simulink subsystem "s8x8_ULA_additive_Noise_Interference"  (R2020b)
settings: Solver=VariableStepAuto  StartTime=0.0  StopTime=10.0  RelTol=1e-3
values from neighbouring files (symbols this model uses):
  fc = 200e6    (= 200000000)    [env_sim_setup.m]
  finf = 0.8*fc    (= 160000000)    [env_sim_setup.m]
  fs = 1e9    (= 1000000000)    [env_sim_setup.m]
  noiseP = 1    [env_sim_setup.m]
  phShftD = (0:1:N-1)*eAngD    [env_sim_setup.m]
  phShftI = (0:1:N-1)*eAngI    [env_sim_setup.m]
  SNR = 1    [env_sim_setup.m]
  sv = sv - 0.0001*1i    [env_sim_setup.m]
undefined symbols (not defined in the file or in its folder): datetime, second
libraries: dspsrcs4 x16, simulink x1
settings Model: Creator=jgentile  LastModifiedBy=jgentile

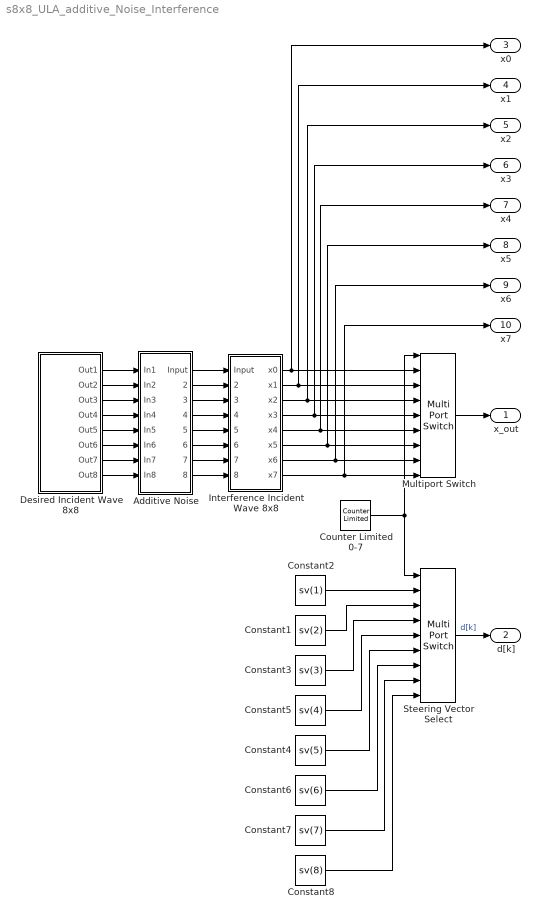
== system s8x8_ULA_additive_Noise_Interference ==
  Additive Noise : Subsystem
  Constant1 : Constant  Value=sv(2)
  Constant2 : Constant  Value=sv(1)
  Constant3 : Constant  Value=sv(3)
  Constant4 : Constant  Value=sv(5)
  Constant5 : Constant  Value=sv(4)
  Constant6 : Constant  Value=sv(6)
  Constant7 : Constant  Value=sv(7)
  Constant8 : Constant  Value=sv(8)
  Counter Limited 0-7 : simulink/Sources/Counter Limited  uplimit=7  tsamp=-1
  Desired Incident Wave 8x8 : Subsystem
  Interference Incident Wave 8x8 : Subsystem
  Multiport Switch : MultiPortSwitch  DataPortOrder=Zero-based contiguous  Inputs=8  zeroidx=on
  Steering Vector Select : MultiPortSwitch  DataPortOrder=Zero-based contiguous  Inputs=8  zeroidx=on
  x_out : Outport
  d[k] : Outport  Port=2
      settings: SignalType=complex
  x0 : Outport  Port=3
  x1 : Outport  Port=4
  x2 : Outport  Port=5
  x3 : Outport  Port=6
  x4 : Outport  Port=7
  x5 : Outport  Port=8
  x6 : Outport  Port=9
  x7 : Outport  Port=10
  wires:
  Constant1/1 -> Steering Vector Select/3
  Constant3/1 -> Steering Vector Select/4
  Multiport Switch/1 -> x_out/1
  Steering Vector Select/1 -> d[k]/1  "d[k]"
  Counter Limited 0-7/1 -> Multiport Switch/1, Steering Vector Select/1
  Constant2/1 -> Steering Vector Select/2
  Desired Incident Wave 8x8/1(Out1) -> Additive Noise/1(In1)
  Desired Incident Wave 8x8/2(Out2) -> Additive Noise/2(In2)
  Desired Incident Wave 8x8/3(Out3) -> Additive Noise/3(In3)
  Additive Noise/1(Input) -> Interference Incident Wave 8x8/1(Input)
  Additive Noise/2(Input1) -> Interference Incident Wave 8x8/2(Input1)
  Additive Noise/3(Input2) -> Interference Incident Wave 8x8/3(Input2)
  Interference Incident Wave 8x8/3(x2) -> x2/1, Multiport Switch/4
  Interference Incident Wave 8x8/2(x1) -> x1/1, Multiport Switch/3
  Interference Incident Wave 8x8/1(x0) -> x0/1, Multiport Switch/2
  Desired Incident Wave 8x8/4(Out4) -> Additive Noise/4(In4)
  Desired Incident Wave 8x8/5(Out5) -> Additive Noise/5(In5)
  Desired Incident Wave 8x8/6(Out6) -> Additive Noise/6(In6)
  Desired Incident Wave 8x8/7(Out7) -> Additive Noise/7(In7)
  Desired Incident Wave 8x8/8(Out8) -> Additive Noise/8(In8)
  Additive Noise/4(Input3) -> Interference Incident Wave 8x8/4(Input3)
  Additive Noise/5(Input4) -> Interference Incident Wave 8x8/5(Input4)
  Additive Noise/6(Input5) -> Interference Incident Wave 8x8/6(Input5)
  Additive Noise/7(Input6) -> Interference Incident Wave 8x8/7(Input6)
  Additive Noise/8(Input7) -> Interference Incident Wave 8x8/8(Input7)
  Interference Incident Wave 8x8/4(x3) -> Multiport Switch/5, x3/1
  Interference Incident Wave 8x8/5(x4) -> Multiport Switch/6, x4/1
  Interference Incident Wave 8x8/6(x5) -> Multiport Switch/7, x5/1
  Interference Incident Wave 8x8/7(x6) -> Multiport Switch/8, x6/1
  Interference Incident Wave 8x8/8(x7) -> Multiport Switch/9, x7/1
  Constant5/1 -> Steering Vector Select/5
  Constant4/1 -> Steering Vector Select/6
  Constant6/1 -> Steering Vector Select/7
  Constant7/1 -> Steering Vector Select/8
  Constant8/1 -> Steering Vector Select/9

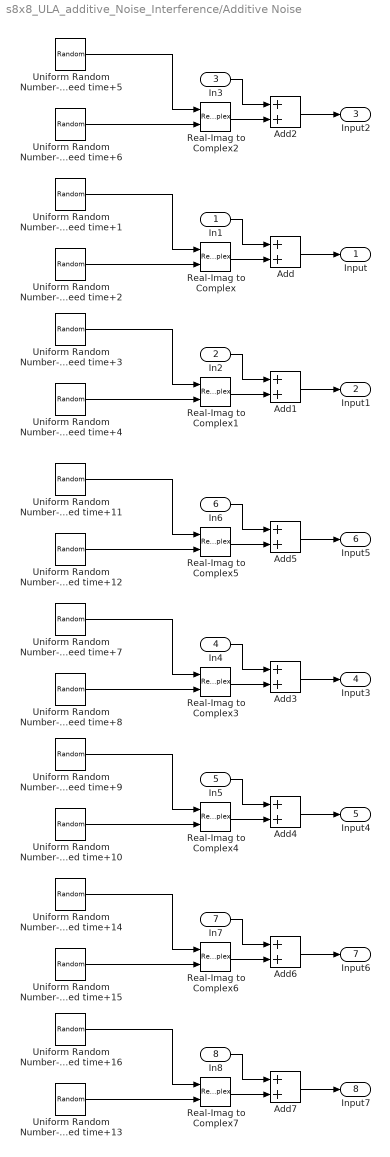
== system s8x8_ULA_additive_Noise_Interference/Additive Noise ==
  In1 : Inport
  In2 : Inport  Port=2
  In3 : Inport  Port=3
  In4 : Inport  Port=4
  In5 : Inport  Port=5
  In6 : Inport  Port=6
  In7 : Inport  Port=7
  In8 : Inport  Port=8
  Add{,1..7} (8 alike) : Sum
  Real-Imag to Complex{,1..7} (8 alike) : RealImagToComplex
  Uniform Random Number- Seed time+1 : UniformRandomNumber  Minimum=-sqrt(SNR*noiseP)  Maximum=sqrt(SNR*noiseP)  Seed=round(second(datetime('now')))+1  SampleTime=1/fs
  Uniform Random Number- Seed time+10 : UniformRandomNumber  Minimum=-sqrt(SNR*noiseP)  Maximum=sqrt(SNR*noiseP)  Seed=round(second(datetime('now')))+4  SampleTime=1/fs
  Uniform Random Number- Seed time+11 : UniformRandomNumber  Minimum=-sqrt(SNR*noiseP)  Maximum=sqrt(SNR*noiseP)  Seed=round(second(datetime('now')))+5  SampleTime=1/fs
  Uniform Random Number- Seed time+12 : UniformRandomNumber  Minimum=-sqrt(SNR*noiseP)  Maximum=sqrt(SNR*noiseP)  Seed=round(second(datetime('now')))+6  SampleTime=1/fs
  Uniform Random Number- Seed time+13 : UniformRandomNumber  Minimum=-sqrt(SNR*noiseP)  Maximum=sqrt(SNR*noiseP)  Seed=round(second(datetime('now')))+4  SampleTime=1/fs
  Uniform Random Number- Seed time+14 : UniformRandomNumber  Minimum=-sqrt(SNR*noiseP)  Maximum=sqrt(SNR*noiseP)  Seed=round(second(datetime('now')))+1  SampleTime=1/fs
  Uniform Random Number- Seed time+15 : UniformRandomNumber  Minimum=-sqrt(SNR*noiseP)  Maximum=sqrt(SNR*noiseP)  Seed=round(second(datetime('now')))+2  SampleTime=1/fs
  Uniform Random Number- Seed time+16 : UniformRandomNumber  Minimum=-sqrt(SNR*noiseP)  Maximum=sqrt(SNR*noiseP)  Seed=round(second(datetime('now')))+3  SampleTime=1/fs
  Uniform Random Number- Seed time+2 : UniformRandomNumber  Minimum=-sqrt(SNR*noiseP)  Maximum=sqrt(SNR*noiseP)  Seed=round(second(datetime('now')))+2  SampleTime=1/fs
  Uniform Random Number- Seed time+3 : UniformRandomNumber  Minimum=-sqrt(SNR*noiseP)  Maximum=sqrt(SNR*noiseP)  Seed=round(second(datetime('now')))+3  SampleTime=1/fs
  Uniform Random Number- Seed time+4 : UniformRandomNumber  Minimum=-sqrt(SNR*noiseP)  Maximum=sqrt(SNR*noiseP)  Seed=round(second(datetime('now')))+4  SampleTime=1/fs
  Uniform Random Number- Seed time+5 : UniformRandomNumber  Minimum=-sqrt(SNR*noiseP)  Maximum=sqrt(SNR*noiseP)  Seed=round(second(datetime('now')))+5  SampleTime=1/fs
  Uniform Random Number- Seed time+6 : UniformRandomNumber  Minimum=-sqrt(SNR*noiseP)  Maximum=sqrt(SNR*noiseP)  Seed=round(second(datetime('now')))+6  SampleTime=1/fs
  Uniform Random Number- Seed time+7 : UniformRandomNumber  Minimum=-sqrt(SNR*noiseP)  Maximum=sqrt(SNR*noiseP)  Seed=round(second(datetime('now')))+1  SampleTime=1/fs
  Uniform Random Number- Seed time+8 : UniformRandomNumber  Minimum=-sqrt(SNR*noiseP)  Maximum=sqrt(SNR*noiseP)  Seed=round(second(datetime('now')))+2  SampleTime=1/fs
  Uniform Random Number- Seed time+9 : UniformRandomNumber  Minimum=-sqrt(SNR*noiseP)  Maximum=sqrt(SNR*noiseP)  Seed=round(second(datetime('now')))+3  SampleTime=1/fs
  Input : Outport
  Input1 : Outport  Port=2
  Input2 : Outport  Port=3
  Input3 : Outport  Port=4
  Input4 : Outport  Port=5
  Input5 : Outport  Port=6
  Input6 : Outport  Port=7
  Input7 : Outport  Port=8
  wires:
  Add/1 -> Input/1
  Uniform Random Number- Seed time+5/1 -> Real-Imag to Complex2/1
  Real-Imag to Complex2/1 -> Add2/2
  Add2/1 -> Input2/1
  Uniform Random Number- Seed time+4/1 -> Real-Imag to Complex1/2
  In3/1 -> Add2/1
  Real-Imag to Complex/1 -> Add/2
  Uniform Random Number- Seed time+3/1 -> Real-Imag to Complex1/1
  In1/1 -> Add/1
  Add1/1 -> Input1/1
  Uniform Random Number- Seed time+2/1 -> Real-Imag to Complex/2
  In2/1 -> Add1/1
  Uniform Random Number- Seed time+1/1 -> Real-Imag to Complex/1
  Uniform Random Number- Seed time+6/1 -> Real-Imag to Complex2/2
  Real-Imag to Complex1/1 -> Add1/2
  Real-Imag to Complex4/1 -> Add4/2
  Uniform Random Number- Seed time+12/1 -> Real-Imag to Complex5/2
  Uniform Random Number- Seed time+7/1 -> Real-Imag to Complex3/1
  In5/1 -> Add4/1
  Uniform Random Number- Seed time+8/1 -> Real-Imag to Complex3/2
  Add4/1 -> Input4/1
  In4/1 -> Add3/1
  Uniform Random Number- Seed time+9/1 -> Real-Imag to Complex4/1
  Real-Imag to Complex3/1 -> Add3/2
  In6/1 -> Add5/1
  Uniform Random Number- Seed time+10/1 -> Real-Imag to Complex4/2
  Add5/1 -> Input5/1
  Real-Imag to Complex5/1 -> Add5/2
  Uniform Random Number- Seed time+11/1 -> Real-Imag to Complex5/1
  Add3/1 -> Input3/1
  Add6/1 -> Input6/1
  Uniform Random Number- Seed time+13/1 -> Real-Imag to Complex7/2
  Real-Imag to Complex6/1 -> Add6/2
  Uniform Random Number- Seed time+16/1 -> Real-Imag to Complex7/1
  In7/1 -> Add6/1
  Add7/1 -> Input7/1
  Uniform Random Number- Seed time+15/1 -> Real-Imag to Complex6/2
  In8/1 -> Add7/1
  Uniform Random Number- Seed time+14/1 -> Real-Imag to Complex6/1
  Real-Imag to Complex7/1 -> Add7/2

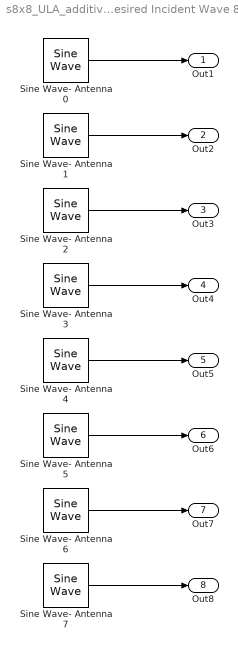
== system s8x8_ULA_additive_Noise_Interference/Desired Incident Wave 8x8 ==
  Sine Wave- Antenna 0 : dspsrcs4/Sine Wave  Amplitude=SNR  Frequency=fc  Phase=phShftD(1)  SampleMode=Discrete  OutComplex=Complex  CompMethod=Trigonometric fcn  TableSize=Speed  SampleTime=1/fs  SamplesPerFrame=1  ResetState=Restart at time zero  OutputFrames=off  dataType=double  wordLen=16  udDataType=sfix(16)  fracBitsMode=Best precision  numFracBits=15  OutDataTypeStr=double  LastOutDataTypeStr=double
  Sine Wave- Antenna 1 : dspsrcs4/Sine Wave  Amplitude=SNR  Frequency=fc  Phase=phShftD(2)  SampleMode=Discrete  OutComplex=Complex  CompMethod=Trigonometric fcn  TableSize=Speed  SampleTime=1/fs  SamplesPerFrame=1  ResetState=Restart at time zero  OutputFrames=off  dataType=double  wordLen=16  udDataType=sfix(16)  fracBitsMode=Best precision  numFracBits=15  OutDataTypeStr=double  LastOutDataTypeStr=double
  Sine Wave- Antenna 2 : dspsrcs4/Sine Wave  Amplitude=SNR  Frequency=fc  Phase=phShftD(3)  SampleMode=Discrete  OutComplex=Complex  CompMethod=Trigonometric fcn  TableSize=Speed  SampleTime=1/fs  SamplesPerFrame=1  ResetState=Restart at time zero  OutputFrames=off  dataType=double  wordLen=16  udDataType=sfix(16)  fracBitsMode=Best precision  numFracBits=15  OutDataTypeStr=double  LastOutDataTypeStr=double
  Sine Wave- Antenna 3 : dspsrcs4/Sine Wave  Amplitude=SNR  Frequency=fc  Phase=phShftD(4)  SampleMode=Discrete  OutComplex=Complex  CompMethod=Trigonometric fcn  TableSize=Speed  SampleTime=1/fs  SamplesPerFrame=1  ResetState=Restart at time zero  OutputFrames=off  dataType=double  wordLen=16  udDataType=sfix(16)  fracBitsMode=Best precision  numFracBits=15  OutDataTypeStr=double  LastOutDataTypeStr=double
  Sine Wave- Antenna 4 : dspsrcs4/Sine Wave  Amplitude=SNR  Frequency=fc  Phase=phShftD(5)  SampleMode=Discrete  OutComplex=Complex  CompMethod=Trigonometric fcn  TableSize=Speed  SampleTime=1/fs  SamplesPerFrame=1  ResetState=Restart at time zero  OutputFrames=off  dataType=double  wordLen=16  udDataType=sfix(16)  fracBitsMode=Best precision  numFracBits=15  OutDataTypeStr=double  LastOutDataTypeStr=double
  Sine Wave- Antenna 5 : dspsrcs4/Sine Wave  Amplitude=SNR  Frequency=fc  Phase=phShftD(6)  SampleMode=Discrete  OutComplex=Complex  CompMethod=Trigonometric fcn  TableSize=Speed  SampleTime=1/fs  SamplesPerFrame=1  ResetState=Restart at time zero  OutputFrames=off  dataType=double  wordLen=16  udDataType=sfix(16)  fracBitsMode=Best precision  numFracBits=15  OutDataTypeStr=double  LastOutDataTypeStr=double
  Sine Wave- Antenna 6 : dspsrcs4/Sine Wave  Amplitude=SNR  Frequency=fc  Phase=phShftD(7)  SampleMode=Discrete  OutComplex=Complex  CompMethod=Trigonometric fcn  TableSize=Speed  SampleTime=1/fs  SamplesPerFrame=1  ResetState=Restart at time zero  OutputFrames=off  dataType=double  wordLen=16  udDataType=sfix(16)  fracBitsMode=Best precision  numFracBits=15  OutDataTypeStr=double  LastOutDataTypeStr=double
  Sine Wave- Antenna 7 : dspsrcs4/Sine Wave  Amplitude=SNR  Frequency=fc  Phase=phShftD(8)  SampleMode=Discrete  OutComplex=Complex  CompMethod=Trigonometric fcn  TableSize=Speed  SampleTime=1/fs  SamplesPerFrame=1  ResetState=Restart at time zero  OutputFrames=off  dataType=double  wordLen=16  udDataType=sfix(16)  fracBitsMode=Best precision  numFracBits=15  OutDataTypeStr=double  LastOutDataTypeStr=double
  Out1 : Outport
  Out2 : Outport  Port=2
  Out3 : Outport  Port=3
  Out4 : Outport  Port=4
  Out5 : Outport  Port=5
  Out6 : Outport  Port=6
  Out7 : Outport  Port=7
  Out8 : Outport  Port=8
  wires:
  Sine Wave- Antenna 1/1 -> Out2/1
  Sine Wave- Antenna 0/1 -> Out1/1
  Sine Wave- Antenna 6/1 -> Out7/1
  Sine Wave- Antenna 7/1 -> Out8/1
  Sine Wave- Antenna 2/1 -> Out3/1
  Sine Wave- Antenna 5/1 -> Out6/1
  Sine Wave- Antenna 4/1 -> Out5/1
  Sine Wave- Antenna 3/1 -> Out4/1

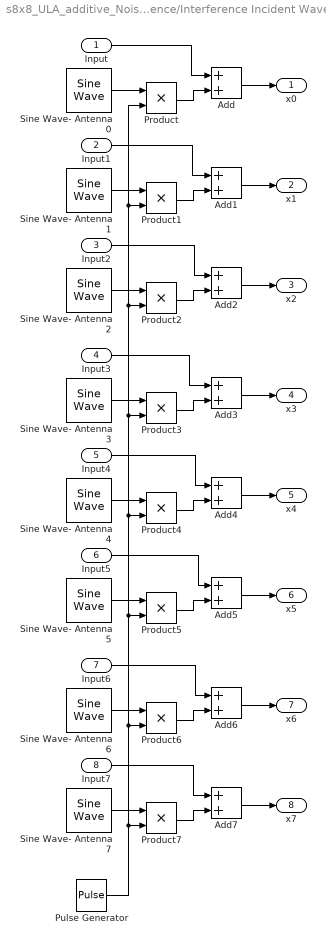
== system s8x8_ULA_additive_Noise_Interference/Interference Incident Wave 8x8 ==
  Input : Inport
  Input1 : Inport  Port=2
  Input2 : Inport  Port=3
  Input3 : Inport  Port=4
  Input4 : Inport  Port=5
  Input5 : Inport  Port=6
  Input6 : Inport  Port=7
  Input7 : Inport  Port=8
  Add{,1..7} (8 alike) : Sum
  Product{,1..7} (8 alike) : Product
  Pulse Generator : DiscretePulseGenerator  Period=10000  PulseWidth=2000  PhaseDelay=3000  SampleTime=1/fs
  Sine Wave- Antenna 0 : dspsrcs4/Sine Wave  Amplitude=4*SNR  Frequency=finf  Phase=phShftI(1)  SampleMode=Discrete  OutComplex=Complex  CompMethod=Trigonometric fcn  TableSize=Speed  SampleTime=1/fs  SamplesPerFrame=1  ResetState=Restart at time zero  OutputFrames=off  dataType=double  wordLen=16  udDataType=sfix(16)  fracBitsMode=Best precision  numFracBits=15  OutDataTypeStr=double  LastOutDataTypeStr=double
  Sine Wave- Antenna 1 : dspsrcs4/Sine Wave  Amplitude=4*SNR  Frequency=finf  Phase=phShftI(2)  SampleMode=Discrete  OutComplex=Complex  CompMethod=Trigonometric fcn  TableSize=Speed  SampleTime=1/fs  SamplesPerFrame=1  ResetState=Restart at time zero  OutputFrames=off  dataType=double  wordLen=16  udDataType=sfix(16)  fracBitsMode=Best precision  numFracBits=15  OutDataTypeStr=double  LastOutDataTypeStr=double
  Sine Wave- Antenna 2 : dspsrcs4/Sine Wave  Amplitude=4*SNR  Frequency=finf  Phase=phShftI(3)  SampleMode=Discrete  OutComplex=Complex  CompMethod=Trigonometric fcn  TableSize=Speed  SampleTime=1/fs  SamplesPerFrame=1  ResetState=Restart at time zero  OutputFrames=off  dataType=double  wordLen=16  udDataType=sfix(16)  fracBitsMode=Best precision  numFracBits=15  OutDataTypeStr=double  LastOutDataTypeStr=double
  Sine Wave- Antenna 3 : dspsrcs4/Sine Wave  Amplitude=4*SNR  Frequency=finf  Phase=phShftI(4)  SampleMode=Discrete  OutComplex=Complex  CompMethod=Trigonometric fcn  TableSize=Speed  SampleTime=1/fs  SamplesPerFrame=1  ResetState=Restart at time zero  OutputFrames=off  dataType=double  wordLen=16  udDataType=sfix(16)  fracBitsMode=Best precision  numFracBits=15  OutDataTypeStr=double  LastOutDataTypeStr=double
  Sine Wave- Antenna 4 : dspsrcs4/Sine Wave  Amplitude=4*SNR  Frequency=finf  Phase=phShftI(5)  SampleMode=Discrete  OutComplex=Complex  CompMethod=Trigonometric fcn  TableSize=Speed  SampleTime=1/fs  SamplesPerFrame=1  ResetState=Restart at time zero  OutputFrames=off  dataType=double  wordLen=16  udDataType=sfix(16)  fracBitsMode=Best precision  numFracBits=15  OutDataTypeStr=double  LastOutDataTypeStr=double
  Sine Wave- Antenna 5 : dspsrcs4/Sine Wave  Amplitude=4*SNR  Frequency=finf  Phase=phShftI(6)  SampleMode=Discrete  OutComplex=Complex  CompMethod=Trigonometric fcn  TableSize=Speed  SampleTime=1/fs  SamplesPerFrame=1  ResetState=Restart at time zero  OutputFrames=off  dataType=double  wordLen=16  udDataType=sfix(16)  fracBitsMode=Best precision  numFracBits=15  OutDataTypeStr=double  LastOutDataTypeStr=double
  Sine Wave- Antenna 6 : dspsrcs4/Sine Wave  Amplitude=4*SNR  Frequency=finf  Phase=phShftI(7)  SampleMode=Discrete  OutComplex=Complex  CompMethod=Trigonometric fcn  TableSize=Speed  SampleTime=1/fs  SamplesPerFrame=1  ResetState=Restart at time zero  OutputFrames=off  dataType=double  wordLen=16  udDataType=sfix(16)  fracBitsMode=Best precision  numFracBits=15  OutDataTypeStr=double  LastOutDataTypeStr=double
  Sine Wave- Antenna 7 : dspsrcs4/Sine Wave  Amplitude=4*SNR  Frequency=finf  Phase=phShftI(8)  SampleMode=Discrete  OutComplex=Complex  CompMethod=Trigonometric fcn  TableSize=Speed  SampleTime=1/fs  SamplesPerFrame=1  ResetState=Restart at time zero  OutputFrames=off  dataType=double  wordLen=16  udDataType=sfix(16)  fracBitsMode=Best precision  numFracBits=15  OutDataTypeStr=double  LastOutDataTypeStr=double
  x0 : Outport
  x1 : Outport  Port=2
  x2 : Outport  Port=3
  x3 : Outport  Port=4
  x4 : Outport  Port=5
  x5 : Outport  Port=6
  x6 : Outport  Port=7
  x7 : Outport  Port=8
  wires:
  Pulse Generator/1 -> Product7/2, Product4/2, Product3/2, Product2/2, Product1/2, Product/2, Product5/2, Product6/2
  Product7/1 -> Add7/2
  Sine Wave- Antenna 7/1 -> Product7/1
  Product6/1 -> Add6/2
  Sine Wave- Antenna 6/1 -> Product6/1
  Product5/1 -> Add5/2
  Sine Wave- Antenna 5/1 -> Product5/1
  Product4/1 -> Add4/2
  Sine Wave- Antenna 4/1 -> Product4/1
  Product3/1 -> Add3/2
  Sine Wave- Antenna 3/1 -> Product3/1
  Product2/1 -> Add2/2
  Sine Wave- Antenna 2/1 -> Product2/1
  Product1/1 -> Add1/2
  Sine Wave- Antenna 1/1 -> Product1/1
  Product/1 -> Add/2
  Sine Wave- Antenna 0/1 -> Product/1
  Input1/1 -> Add1/1
  Add1/1 -> x1/1
  Add2/1 -> x2/1
  Input2/1 -> Add2/1
  Add/1 -> x0/1
  Input/1 -> Add/1
  Input3/1 -> Add3/1
  Add3/1 -> x3/1
  Input5/1 -> Add5/1
  Add5/1 -> x5/1
  Add4/1 -> x4/1
  Input4/1 -> Add4/1
  Input6/1 -> Add6/1
  Add6/1 -> x6/1
  Add7/1 -> x7/1
  Input7/1 -> Add7/1
